simulink model "Distribution_v2"  (Simulink 7.9)
settings: Solver=VariableStepDiscrete  StartTime=0.0  StopTime=1000  RelTol=1e-3
libraries: simeventslib x35
(part 2 of 6)

== system Distribution_v2/Customer_6 ==
  Commodity_44 : Subsystem  mask{Mean=2000/49, AttributeValue=[6  18  22   1]|6|1|1}
      mask prompts: Mean "Frequency"; AttributeValue "Attributes"
  Commodity_45 : Subsystem  mask{Mean=2000/472, AttributeValue=[6  18   2   0]|6|2|1}
      mask prompts: Mean "Frequency"; AttributeValue "Attributes"
  Commodity_46 : Subsystem  mask{Mean=2000/118, AttributeValue=[6  18  22   5]|6|5|1}
      mask prompts: Mean "Frequency"; AttributeValue "Attributes"
  Commodity_47 : Subsystem  mask{Mean=2000/411, AttributeValue=[6  18  20   7]|6|7|1}
      mask prompts: Mean "Frequency"; AttributeValue "Attributes"
  Commodity_48 : Subsystem  mask{Mean=2000/22, AttributeValue=[6  18  20   8]|6|8|1}
      mask prompts: Mean "Frequency"; AttributeValue "Attributes"
  Commodity_49 : Subsystem  mask{Mean=2000/325, AttributeValue=[6  18   9   0]|6|9|1}
      mask prompts: Mean "Frequency"; AttributeValue "Attributes"
  Commodity_50 : Subsystem  mask{Mean=2000/274, AttributeValue=[6  18  22  12]|6|12|1}
      mask prompts: Mean "Frequency"; AttributeValue "Attributes"
  Commodity_51 : Subsystem  mask{Mean=2000/373, AttributeValue=[6  18  22  13]|6|13|1}
      mask prompts: Mean "Frequency"; AttributeValue "Attributes"
  Commodity_52 : Subsystem  mask{Mean=2000/344, AttributeValue=[6  18  20  14]|6|14|1}
      mask prompts: Mean "Frequency"; AttributeValue "Attributes"
  Commodity_53 : Subsystem  mask{Mean=2000/185, AttributeValue=[6  18  20  15]|6|15|1}
      mask prompts: Mean "Frequency"; AttributeValue "Attributes"
  Entity Sink : EntitySink
  Get Attribute : GetAttribute  AttributeName=Origin|Destination|Start  AttributeMissing=Error|Error|Error  AttributeDefaultValue=1|1|1  AttributeTreatAsVector=1|1|1  AttributeSendTiming=After entity departure|After entity departure|After entity departure  EvaluatedDefaultAttributeValue={[];[];[]}
      settings: OutputPortMap=o1,o2,o3
  Get Attribute1 : GetAttribute  AttributeName=Route  EvaluatedDefaultAttributeValue={[]}
      settings: OutputPortMap=o1
  IN_Commodity : PathCombiner  NumberInputPorts=10
  IN_Shipment : PathCombiner  NumberInputPorts=1
  Lookup : Constant  Value=[18]
  MATLAB Function : MATLAB Function  TreatAsAtomicUnit=on
  Mux : Mux  Inputs=3
  Node_ID : Constant  Value=6
  OUT_Shipment : OutputSwitch  NumberOutputPorts=1  SwitchingCriterion=From signal port p  AttributeName=Customer
  Shipment_Metrics : simeventslib/SimEvents Sinks/Discrete Event Signal to Workspace  VariableName=Customer_6  SaveFormat=Structure With Time  isMonitorOnly=off  isRecordIC=off
  Single Server : SingleServer  ServiceTime=0
  Timed to Evnt Signal : TimedToEventSignal
  Timed to Evnt Signal1 : TimedToEventSignal
  IN_Shipment_1 : PMIOPort  Port=1  Side=Left
  OUT_Shipment_1 : PMIOPort  Port=2  Side=Right
  wires:
  Timed to Evnt Signal1/1 -> MATLAB Function/3(lookup)
  Lookup/1 -> Timed to Evnt Signal1/1
  Timed to Evnt Signal/1 -> MATLAB Function/2(current)
  Get Attribute1/1 -> MATLAB Function/1(route)
  MATLAB Function/1(next) -> OUT_Shipment/1
  Node_ID/1 -> Timed to Evnt Signal/1
  Mux/1 -> Shipment_Metrics/1
  Get Attribute/3 -> Mux/3
  Get Attribute/2 -> Mux/2
  Get Attribute/1 -> Mux/1
  connections:
  Single Server/RConn1 -- OUT_Shipment/LConn1
  Get Attribute1/RConn1 -- Single Server/LConn1
  IN_Commodity/RConn1 -- Get Attribute1/LConn1
  Get Attribute/LConn1 -- IN_Shipment/RConn1
  Entity Sink/LConn1 -- Get Attribute/RConn1
  IN_Shipment/LConn1 -- IN_Shipment_1/RConn1
  OUT_Shipment/RConn1 -- OUT_Shipment_1/RConn1
  Commodity_44/RConn1 -- IN_Commodity/LConn1
  Commodity_45/RConn1 -- IN_Commodity/LConn2
  Commodity_46/RConn1 -- IN_Commodity/LConn3
  Commodity_47/RConn1 -- IN_Commodity/LConn4
  Commodity_48/RConn1 -- IN_Commodity/LConn5
  Commodity_49/RConn1 -- IN_Commodity/LConn6
  Commodity_50/RConn1 -- IN_Commodity/LConn7
  Commodity_51/RConn1 -- IN_Commodity/LConn8
  Commodity_52/RConn1 -- IN_Commodity/LConn9
  Commodity_53/RConn1 -- IN_Commodity/LConn10

== system Distribution_v2/Customer_7 ==
  Commodity_54 : Subsystem  mask{Mean=2000/465, AttributeValue=[7  20   3   0]|7|3|1}
      mask prompts: Mean "Frequency"; AttributeValue "Attributes"
  Commodity_55 : Subsystem  mask{Mean=2000/218, AttributeValue=[7  20  22   5]|7|5|1}
      mask prompts: Mean "Frequency"; AttributeValue "Attributes"
  Commodity_56 : Subsystem  mask{Mean=2000/154, AttributeValue=[7  20  18   6]|7|6|1}
      mask prompts: Mean "Frequency"; AttributeValue "Attributes"
  Commodity_57 : Subsystem  mask{Mean=2000/406, AttributeValue=[7  20  22  13]|7|13|1}
      mask prompts: Mean "Frequency"; AttributeValue "Attributes"
  Commodity_58 : Subsystem  mask{Mean=2000/470, AttributeValue=[7  20  15   0]|7|15|1}
      mask prompts: Mean "Frequency"; AttributeValue "Attributes"
  Entity Sink : EntitySink
  Get Attribute : GetAttribute  AttributeName=Origin|Destination|Start  AttributeMissing=Error|Error|Error  AttributeDefaultValue=1|1|1  AttributeTreatAsVector=1|1|1  AttributeSendTiming=After entity departure|After entity departure|After entity departure  EvaluatedDefaultAttributeValue={[];[];[]}
      settings: OutputPortMap=o1,o2,o3
  Get Attribute1 : GetAttribute  AttributeName=Route  EvaluatedDefaultAttributeValue={[]}
      settings: OutputPortMap=o1
  IN_Commodity : PathCombiner  NumberInputPorts=5
  IN_Shipment : PathCombiner  NumberInputPorts=1
  Lookup : Constant  Value=[20]
  MATLAB Function : MATLAB Function  TreatAsAtomicUnit=on
  Mux : Mux  Inputs=3
  Node_ID : Constant  Value=7
  OUT_Shipment : OutputSwitch  NumberOutputPorts=1  SwitchingCriterion=From signal port p  AttributeName=Customer
  Shipment_Metrics : simeventslib/SimEvents Sinks/Discrete Event Signal to Workspace  VariableName=Customer_7  SaveFormat=Structure With Time  isMonitorOnly=off  isRecordIC=off
  Single Server : SingleServer  ServiceTime=0
  Timed to Evnt Signal : TimedToEventSignal
  Timed to Evnt Signal1 : TimedToEventSignal
  IN_Shipment_1 : PMIOPort  Port=1  Side=Left
  OUT_Shipment_1 : PMIOPort  Port=2  Side=Right
  wires:
  Timed to Evnt Signal1/1 -> MATLAB Function/3(lookup)
  Lookup/1 -> Timed to Evnt Signal1/1
  Timed to Evnt Signal/1 -> MATLAB Function/2(current)
  Get Attribute1/1 -> MATLAB Function/1(route)
  MATLAB Function/1(next) -> OUT_Shipment/1
  Node_ID/1 -> Timed to Evnt Signal/1
  Mux/1 -> Shipment_Metrics/1
  Get Attribute/3 -> Mux/3
  Get Attribute/2 -> Mux/2
  Get Attribute/1 -> Mux/1
  connections:
  Single Server/RConn1 -- OUT_Shipment/LConn1
  Get Attribute1/RConn1 -- Single Server/LConn1
  IN_Commodity/RConn1 -- Get Attribute1/LConn1
  Get Attribute/LConn1 -- IN_Shipment/RConn1
  Entity Sink/LConn1 -- Get Attribute/RConn1
  IN_Shipment/LConn1 -- IN_Shipment_1/RConn1
  OUT_Shipment/RConn1 -- OUT_Shipment_1/RConn1
  Commodity_54/RConn1 -- IN_Commodity/LConn1
  Commodity_55/RConn1 -- IN_Commodity/LConn2
  Commodity_56/RConn1 -- IN_Commodity/LConn3
  Commodity_57/RConn1 -- IN_Commodity/LConn4
  Commodity_58/RConn1 -- IN_Commodity/LConn5

== system Distribution_v2/Customer_8 ==
  Commodity_59 : Subsystem  mask{Mean=2000/151, AttributeValue=[8  20  22   5]|8|5|1}
      mask prompts: Mean "Frequency"; AttributeValue "Attributes"
  Commodity_60 : Subsystem  mask{Mean=2000/116, AttributeValue=[8  20  18   6]|8|6|1}
      mask prompts: Mean "Frequency"; AttributeValue "Attributes"
  Commodity_61 : Subsystem  mask{Mean=2000/113, AttributeValue=[8  20  18   9]|8|9|1}
      mask prompts: Mean "Frequency"; AttributeValue "Attributes"
  Commodity_62 : Subsystem  mask{Mean=2000/114, AttributeValue=[8  20  22  10]|8|10|1}
      mask prompts: Mean "Frequency"; AttributeValue "Attributes"
  Commodity_63 : Subsystem  mask{Mean=2000/156, AttributeValue=[8  20  11   0]|8|11|1}
      mask prompts: Mean "Frequency"; AttributeValue "Attributes"
  Commodity_64 : Subsystem  mask{Mean=2000/93, AttributeValue=[8  20  22  13]|8|13|1}
      mask prompts: Mean "Frequency"; AttributeValue "Attributes"
  Entity Sink : EntitySink
  Get Attribute : GetAttribute  AttributeName=Origin|Destination|Start  AttributeMissing=Error|Error|Error  AttributeDefaultValue=1|1|1  AttributeTreatAsVector=1|1|1  AttributeSendTiming=After entity departure|After entity departure|After entity departure  EvaluatedDefaultAttributeValue={[];[];[]}
      settings: OutputPortMap=o1,o2,o3
  Get Attribute1 : GetAttribute  AttributeName=Route  EvaluatedDefaultAttributeValue={[]}
      settings: OutputPortMap=o1
  IN_Commodity : PathCombiner  NumberInputPorts=6
  IN_Shipment : PathCombiner  NumberInputPorts=1
  Lookup : Constant  Value=[20]
  MATLAB Function : MATLAB Function  TreatAsAtomicUnit=on
  Mux : Mux  Inputs=3
  Node_ID : Constant  Value=8
  OUT_Shipment : OutputSwitch  NumberOutputPorts=1  SwitchingCriterion=From signal port p  AttributeName=Customer
  Shipment_Metrics : simeventslib/SimEvents Sinks/Discrete Event Signal to Workspace  VariableName=Customer_8  SaveFormat=Structure With Time  isMonitorOnly=off  isRecordIC=off
  Single Server : SingleServer  ServiceTime=0
  Timed to Evnt Signal : TimedToEventSignal
  Timed to Evnt Signal1 : TimedToEventSignal
  IN_Shipment_1 : PMIOPort  Port=1  Side=Left
  OUT_Shipment_1 : PMIOPort  Port=2  Side=Right
  wires:
  Timed to Evnt Signal1/1 -> MATLAB Function/3(lookup)
  Lookup/1 -> Timed to Evnt Signal1/1
  Timed to Evnt Signal/1 -> MATLAB Function/2(current)
  Get Attribute1/1 -> MATLAB Function/1(route)
  MATLAB Function/1(next) -> OUT_Shipment/1
  Node_ID/1 -> Timed to Evnt Signal/1
  Mux/1 -> Shipment_Metrics/1
  Get Attribute/3 -> Mux/3
  Get Attribute/2 -> Mux/2
  Get Attribute/1 -> Mux/1
  connections:
  Single Server/RConn1 -- OUT_Shipment/LConn1
  Get Attribute1/RConn1 -- Single Server/LConn1
  IN_Commodity/RConn1 -- Get Attribute1/LConn1
  Get Attribute/LConn1 -- IN_Shipment/RConn1
  Entity Sink/LConn1 -- Get Attribute/RConn1
  IN_Shipment/LConn1 -- IN_Shipment_1/RConn1
  OUT_Shipment/RConn1 -- OUT_Shipment_1/RConn1
  Commodity_59/RConn1 -- IN_Commodity/LConn1
  Commodity_60/RConn1 -- IN_Commodity/LConn2
  Commodity_61/RConn1 -- IN_Commodity/LConn3
  Commodity_62/RConn1 -- IN_Commodity/LConn4
  Commodity_63/RConn1 -- IN_Commodity/LConn5
  Commodity_64/RConn1 -- IN_Commodity/LConn6

== system Distribution_v2/Customer_9 ==
  Commodity_65 : Subsystem  mask{Mean=2000/56, AttributeValue=[9  18  22   1]|9|1|1}
      mask prompts: Mean "Frequency"; AttributeValue "Attributes"
  Commodity_66 : Subsystem  mask{Mean=2000/205, AttributeValue=[9  18   2   0]|9|2|1}
      mask prompts: Mean "Frequency"; AttributeValue "Attributes"
  Commodity_67 : Subsystem  mask{Mean=2000/302, AttributeValue=[9  18   4   0]|9|4|1}
      mask prompts: Mean "Frequency"; AttributeValue "Attributes"
  Commodity_68 : Subsystem  mask{Mean=2000/59, AttributeValue=[9  18   6   0]|9|6|1}
      mask prompts: Mean "Frequency"; AttributeValue "Attributes"
  Commodity_69 : Subsystem  mask{Mean=2000/160, AttributeValue=[9  18  20   7]|9|7|1}
      mask prompts: Mean "Frequency"; AttributeValue "Attributes"
  Commodity_70 : Subsystem  mask{Mean=2000/254, AttributeValue=[9  18  20   8]|9|8|1}
      mask prompts: Mean "Frequency"; AttributeValue "Attributes"
  Commodity_71 : Subsystem  mask{Mean=2000/132, AttributeValue=[9  18  22  10]|9|10|1}
      mask prompts: Mean "Frequency"; AttributeValue "Attributes"
  Commodity_72 : Subsystem  mask{Mean=2000/465, AttributeValue=[9  18  22  12]|9|12|1}
      mask prompts: Mean "Frequency"; AttributeValue "Attributes"
  Commodity_73 : Subsystem  mask{Mean=2000/290, AttributeValue=[9  18  20  14]|9|14|1}
      mask prompts: Mean "Frequency"; AttributeValue "Attributes"
  Commodity_74 : Subsystem  mask{Mean=2000/230, AttributeValue=[9  18  20  15]|9|15|1}
      mask prompts: Mean "Frequency"; AttributeValue "Attributes"
  Entity Sink : EntitySink
  Get Attribute : GetAttribute  AttributeName=Origin|Destination|Start  AttributeMissing=Error|Error|Error  AttributeDefaultValue=1|1|1  AttributeTreatAsVector=1|1|1  AttributeSendTiming=After entity departure|After entity departure|After entity departure  EvaluatedDefaultAttributeValue={[];[];[]}
      settings: OutputPortMap=o1,o2,o3
  Get Attribute1 : GetAttribute  AttributeName=Route  EvaluatedDefaultAttributeValue={[]}
      settings: OutputPortMap=o1
  IN_Commodity : PathCombiner  NumberInputPorts=10
  IN_Shipment : PathCombiner  NumberInputPorts=1
  Lookup : Constant  Value=[18]
  MATLAB Function : MATLAB Function  TreatAsAtomicUnit=on
  Mux : Mux  Inputs=3
  Node_ID : Constant  Value=9
  OUT_Shipment : OutputSwitch  NumberOutputPorts=1  SwitchingCriterion=From signal port p  AttributeName=Customer
  Shipment_Metrics : simeventslib/SimEvents Sinks/Discrete Event Signal to Workspace  VariableName=Customer_9  SaveFormat=Structure With Time  isMonitorOnly=off  isRecordIC=off
  Single Server : SingleServer  ServiceTime=0
  Timed to Evnt Signal : TimedToEventSignal
  Timed to Evnt Signal1 : TimedToEventSignal
  IN_Shipment_1 : PMIOPort  Port=1  Side=Left
  OUT_Shipment_1 : PMIOPort  Port=2  Side=Right
  wires:
  Timed to Evnt Signal1/1 -> MATLAB Function/3(lookup)
  Lookup/1 -> Timed to Evnt Signal1/1
  Timed to Evnt Signal/1 -> MATLAB Function/2(current)
  Get Attribute1/1 -> MATLAB Function/1(route)
  MATLAB Function/1(next) -> OUT_Shipment/1
  Node_ID/1 -> Timed to Evnt Signal/1
  Mux/1 -> Shipment_Metrics/1
  Get Attribute/3 -> Mux/3
  Get Attribute/2 -> Mux/2
  Get Attribute/1 -> Mux/1
  connections:
  Single Server/RConn1 -- OUT_Shipment/LConn1
  Get Attribute1/RConn1 -- Single Server/LConn1
  IN_Commodity/RConn1 -- Get Attribute1/LConn1
  Get Attribute/LConn1 -- IN_Shipment/RConn1
  Entity Sink/LConn1 -- Get Attribute/RConn1
  IN_Shipment/LConn1 -- IN_Shipment_1/RConn1
  OUT_Shipment/RConn1 -- OUT_Shipment_1/RConn1
  Commodity_65/RConn1 -- IN_Commodity/LConn1
  Commodity_66/RConn1 -- IN_Commodity/LConn2
  Commodity_67/RConn1 -- IN_Commodity/LConn3
  Commodity_68/RConn1 -- IN_Commodity/LConn4
  Commodity_69/RConn1 -- IN_Commodity/LConn5
  Commodity_70/RConn1 -- IN_Commodity/LConn6
  Commodity_71/RConn1 -- IN_Commodity/LConn7
  Commodity_72/RConn1 -- IN_Commodity/LConn8
  Commodity_73/RConn1 -- IN_Commodity/LConn9
  Commodity_74/RConn1 -- IN_Commodity/LConn10

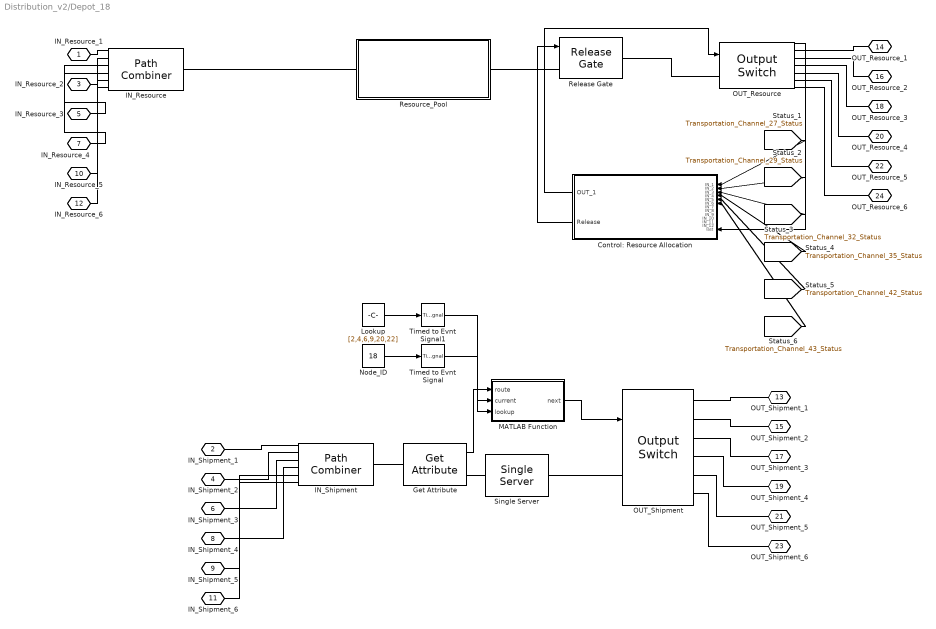
== system Distribution_v2/Depot_18 ==
  Control: Resource Allocation : MATLAB Function  TreatAsAtomicUnit=on
  Get Attribute : GetAttribute  AttributeName=Route  EvaluatedDefaultAttributeValue={[]}
      settings: OutputPortMap=o1
  IN_Resource : PathCombiner  NumberInputPorts=6
  IN_Shipment : PathCombiner  NumberInputPorts=6
  Lookup : Constant  Value=[2,4,6,9,20,22]
  MATLAB Function : MATLAB Function  TreatAsAtomicUnit=on
  Node_ID : Constant  Value=18
  OUT_Resource : OutputSwitch  NumberOutputPorts=6  SwitchingCriterion=From signal port p  InitialSeed=57769  StatLastDeparturePort=on
      settings: OutputPortMap=o3
  OUT_Shipment : OutputSwitch  NumberOutputPorts=6  SwitchingCriterion=From signal port p  AttributeName=Customer
  Release Gate : ReleaseGate  OpenGateUpon=Function call from port fcn
  Resource_Pool : Subsystem  mask{Quantity=6}
      mask prompts: Quantity "How many entities in resource pool?"
  Single Server : SingleServer  ServiceTime=0
  Timed to Evnt Signal : TimedToEventSignal
  Timed to Evnt Signal1 : TimedToEventSignal
  IN_Resource_1 : PMIOPort  Port=1  Side=Left
  IN_Shipment_1 : PMIOPort  Port=2  Side=Left
  IN_Resource_2 : PMIOPort  Port=3  Side=Left
  IN_Shipment_2 : PMIOPort  Port=4  Side=Left
  IN_Resource_3 : PMIOPort  Port=5  Side=Left
  IN_Shipment_3 : PMIOPort  Port=6  Side=Left
  IN_Resource_4 : PMIOPort  Port=7  Side=Left
  IN_Shipment_4 : PMIOPort  Port=8  Side=Left
  IN_Shipment_5 : PMIOPort  Port=9  Side=Left
  IN_Resource_5 : PMIOPort  Port=10  Side=Left
  IN_Shipment_6 : PMIOPort  Port=11  Side=Left
  IN_Resource_6 : PMIOPort  Port=12  Side=Left
  OUT_Shipment_1 : PMIOPort  Port=13  Side=Right
  OUT_Resource_1 : PMIOPort  Port=14  Side=Right
  OUT_Shipment_2 : PMIOPort  Port=15  Side=Right
  OUT_Resource_2 : PMIOPort  Port=16  Side=Right
  OUT_Shipment_3 : PMIOPort  Port=17  Side=Right
  OUT_Resource_3 : PMIOPort  Port=18  Side=Right
  OUT_Shipment_4 : PMIOPort  Port=19  Side=Right
  OUT_Resource_4 : PMIOPort  Port=20  Side=Right
  OUT_Shipment_5 : PMIOPort  Port=21  Side=Right
  OUT_Resource_5 : PMIOPort  Port=22  Side=Right
  OUT_Shipment_6 : PMIOPort  Port=23  Side=Right
  OUT_Resource_6 : PMIOPort  Port=24  Side=Right
  wires:
  OUT_Resource/1 -> Control: Resource Allocation/13(last)
  Control: Resource Allocation/2(Release) -> Release Gate/1
  Control: Resource Allocation/1(OUT_1) -> OUT_Resource/1
  Timed to Evnt Signal1/1 -> MATLAB Function/3(lookup)
  Lookup/1 -> Timed to Evnt Signal1/1
  Timed to Evnt Signal/1 -> MATLAB Function/2(current)
  Get Attribute/1 -> MATLAB Function/1(route)
  MATLAB Function/1(next) -> OUT_Shipment/1
  Node_ID/1 -> Timed to Evnt Signal/1
  [Transportation_Channel_27_Status] -> Control: Resource Allocation/1(IN_1)
  [Transportation_Channel_29_Status] -> Control: Resource Allocation/2(IN_2)
  [Transportation_Channel_32_Status] -> Control: Resource Allocation/3(IN_3)
  [Transportation_Channel_35_Status] -> Control: Resource Allocation/4(IN_4)
  [Transportation_Channel_42_Status] -> Control: Resource Allocation/5(IN_5)
  [Transportation_Channel_43_Status] -> Control: Resource Allocation/6(IN_6)
  connections:
  Release Gate/RConn1 -- OUT_Resource/LConn1
  Resource_Pool/LConn1 -- Release Gate/LConn1
  Single Server/RConn1 -- OUT_Shipment/LConn1
  Get Attribute/RConn1 -- Single Server/LConn1
  IN_Shipment/RConn1 -- Get Attribute/LConn1
  Resource_Pool/RConn1 -- IN_Resource/RConn1
  IN_Resource/LConn1 -- IN_Resource_1/RConn1
  IN_Resource/LConn2 -- IN_Resource_2/RConn1
  IN_Resource/LConn3 -- IN_Resource_3/RConn1
  IN_Resource/LConn4 -- IN_Resource_4/RConn1
  IN_Resource/LConn5 -- IN_Resource_5/RConn1
  IN_Resource/LConn6 -- IN_Resource_6/RConn1
  OUT_Resource/RConn1 -- OUT_Resource_1/RConn1
  OUT_Resource/RConn2 -- OUT_Resource_2/RConn1
  OUT_Resource/RConn3 -- OUT_Resource_3/RConn1
  OUT_Resource/RConn4 -- OUT_Resource_4/RConn1
  OUT_Resource/RConn5 -- OUT_Resource_5/RConn1
  OUT_Resource/RConn6 -- OUT_Resource_6/RConn1
  IN_Shipment/LConn1 -- IN_Shipment_1/RConn1
  IN_Shipment/LConn2 -- IN_Shipment_2/RConn1
  IN_Shipment/LConn3 -- IN_Shipment_3/RConn1
  IN_Shipment/LConn4 -- IN_Shipment_4/RConn1
  IN_Shipment/LConn5 -- IN_Shipment_5/RConn1
  IN_Shipment/LConn6 -- IN_Shipment_6/RConn1
  OUT_Shipment/RConn1 -- OUT_Shipment_1/RConn1
  OUT_Shipment/RConn2 -- OUT_Shipment_2/RConn1
  OUT_Shipment/RConn3 -- OUT_Shipment_3/RConn1
  OUT_Shipment/RConn4 -- OUT_Shipment_4/RConn1
  OUT_Shipment/RConn5 -- OUT_Shipment_5/RConn1
  OUT_Shipment/RConn6 -- OUT_Shipment_6/RConn1

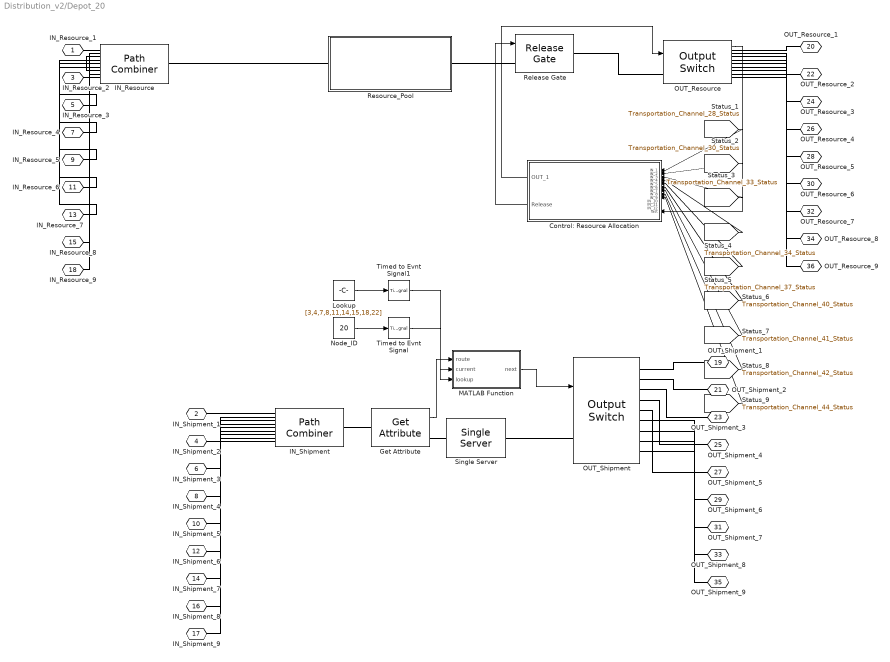
== system Distribution_v2/Depot_20 ==
  Control: Resource Allocation : MATLAB Function  TreatAsAtomicUnit=on
  Get Attribute : GetAttribute  AttributeName=Route  EvaluatedDefaultAttributeValue={[]}
      settings: OutputPortMap=o1
  IN_Resource : PathCombiner  NumberInputPorts=9
  IN_Shipment : PathCombiner  NumberInputPorts=9
  Lookup : Constant  Value=[3,4,7,8,11,14,15,18,22]
  MATLAB Function : MATLAB Function  TreatAsAtomicUnit=on
  Node_ID : Constant  Value=20
  OUT_Resource : OutputSwitch  NumberOutputPorts=9  SwitchingCriterion=From signal port p  InitialSeed=57769  StatLastDeparturePort=on
      settings: OutputPortMap=o3
  OUT_Shipment : OutputSwitch  NumberOutputPorts=9  SwitchingCriterion=From signal port p  AttributeName=Customer
  Release Gate : ReleaseGate  OpenGateUpon=Function call from port fcn
  Resource_Pool : Subsystem  mask{Quantity=6}
      mask prompts: Quantity "How many entities in resource pool?"
  Single Server : SingleServer  ServiceTime=0
  Timed to Evnt Signal : TimedToEventSignal
  Timed to Evnt Signal1 : TimedToEventSignal
  IN_Resource_1 : PMIOPort  Port=1  Side=Left
  IN_Shipment_1 : PMIOPort  Port=2  Side=Left
  IN_Resource_2 : PMIOPort  Port=3  Side=Left
  IN_Shipment_2 : PMIOPort  Port=4  Side=Left
  IN_Resource_3 : PMIOPort  Port=5  Side=Left
  IN_Shipment_3 : PMIOPort  Port=6  Side=Left
  IN_Resource_4 : PMIOPort  Port=7  Side=Left
  IN_Shipment_4 : PMIOPort  Port=8  Side=Left
  IN_Resource_5 : PMIOPort  Port=9  Side=Left
  IN_Shipment_5 : PMIOPort  Port=10  Side=Left
  IN_Resource_6 : PMIOPort  Port=11  Side=Left
  IN_Shipment_6 : PMIOPort  Port=12  Side=Left
  IN_Resource_7 : PMIOPort  Port=13  Side=Left
  IN_Shipment_7 : PMIOPort  Port=14  Side=Left
  IN_Resource_8 : PMIOPort  Port=15  Side=Left
  IN_Shipment_8 : PMIOPort  Port=16  Side=Left
  IN_Shipment_9 : PMIOPort  Port=17  Side=Left
  IN_Resource_9 : PMIOPort  Port=18  Side=Left
  OUT_Shipment_1 : PMIOPort  Port=19  Side=Right
  OUT_Resource_1 : PMIOPort  Port=20  Side=Right
  OUT_Shipment_2 : PMIOPort  Port=21  Side=Right
  OUT_Resource_2 : PMIOPort  Port=22  Side=Right
  OUT_Shipment_3 : PMIOPort  Port=23  Side=Right
  OUT_Resource_3 : PMIOPort  Port=24  Side=Right
  OUT_Shipment_4 : PMIOPort  Port=25  Side=Right
  OUT_Resource_4 : PMIOPort  Port=26  Side=Right
  OUT_Shipment_5 : PMIOPort  Port=27  Side=Right
  OUT_Resource_5 : PMIOPort  Port=28  Side=Right
  OUT_Shipment_6 : PMIOPort  Port=29  Side=Right
  OUT_Resource_6 : PMIOPort  Port=30  Side=Right
  OUT_Shipment_7 : PMIOPort  Port=31  Side=Right
  OUT_Resource_7 : PMIOPort  Port=32  Side=Right
  OUT_Shipment_8 : PMIOPort  Port=33  Side=Right
  OUT_Resource_8 : PMIOPort  Port=34  Side=Right
  OUT_Shipment_9 : PMIOPort  Port=35  Side=Right
  OUT_Resource_9 : PMIOPort  Port=36  Side=Right
  wires:
  OUT_Resource/1 -> Control: Resource Allocation/13(last)
  Control: Resource Allocation/2(Release) -> Release Gate/1
  Control: Resource Allocation/1(OUT_1) -> OUT_Resource/1
  Timed to Evnt Signal1/1 -> MATLAB Function/3(lookup)
  Lookup/1 -> Timed to Evnt Signal1/1
  Timed to Evnt Signal/1 -> MATLAB Function/2(current)
  Get Attribute/1 -> MATLAB Function/1(route)
  MATLAB Function/1(next) -> OUT_Shipment/1
  Node_ID/1 -> Timed to Evnt Signal/1
  [Transportation_Channel_28_Status] -> Control: Resource Allocation/1(IN_1)
  [Transportation_Channel_30_Status] -> Control: Resource Allocation/2(IN_2)
  [Transportation_Channel_33_Status] -> Control: Resource Allocation/3(IN_3)
  [Transportation_Channel_34_Status] -> Control: Resource Allocation/4(IN_4)
  [Transportation_Channel_37_Status] -> Control: Resource Allocation/5(IN_5)
  [Transportation_Channel_40_Status] -> Control: Resource Allocation/6(IN_6)
  [Transportation_Channel_41_Status] -> Control: Resource Allocation/7(IN_7)
  [Transportation_Channel_42_Status] -> Control: Resource Allocation/8(IN_8)
  [Transportation_Channel_44_Status] -> Control: Resource Allocation/9(IN_9)
  connections:
  Release Gate/RConn1 -- OUT_Resource/LConn1
  Resource_Pool/LConn1 -- Release Gate/LConn1
  Single Server/RConn1 -- OUT_Shipment/LConn1
  Get Attribute/RConn1 -- Single Server/LConn1
  IN_Shipment/RConn1 -- Get Attribute/LConn1
  Resource_Pool/RConn1 -- IN_Resource/RConn1
  IN_Resource/LConn1 -- IN_Resource_1/RConn1
  IN_Resource/LConn2 -- IN_Resource_2/RConn1
  IN_Resource/LConn3 -- IN_Resource_3/RConn1
  IN_Resource/LConn4 -- IN_Resource_4/RConn1
  IN_Resource/LConn5 -- IN_Resource_5/RConn1
  IN_Resource/LConn6 -- IN_Resource_6/RConn1
  IN_Resource/LConn7 -- IN_Resource_7/RConn1
  IN_Resource/LConn8 -- IN_Resource_8/RConn1
  IN_Resource/LConn9 -- IN_Resource_9/RConn1
  OUT_Resource/RConn1 -- OUT_Resource_1/RConn1
  OUT_Resource/RConn2 -- OUT_Resource_2/RConn1
  OUT_Resource/RConn3 -- OUT_Resource_3/RConn1
  OUT_Resource/RConn4 -- OUT_Resource_4/RConn1
  OUT_Resource/RConn5 -- OUT_Resource_5/RConn1
  OUT_Resource/RConn6 -- OUT_Resource_6/RConn1
  OUT_Resource/RConn7 -- OUT_Resource_7/RConn1
  OUT_Resource/RConn8 -- OUT_Resource_8/RConn1
  OUT_Resource/RConn9 -- OUT_Resource_9/RConn1
  IN_Shipment/LConn1 -- IN_Shipment_1/RConn1
  IN_Shipment/LConn2 -- IN_Shipment_2/RConn1
  IN_Shipment/LConn3 -- IN_Shipment_3/RConn1
  IN_Shipment/LConn4 -- IN_Shipment_4/RConn1
  IN_Shipment/LConn5 -- IN_Shipment_5/RConn1
  IN_Shipment/LConn6 -- IN_Shipment_6/RConn1
  IN_Shipment/LConn7 -- IN_Shipment_7/RConn1
  IN_Shipment/LConn8 -- IN_Shipment_8/RConn1
  IN_Shipment/LConn9 -- IN_Shipment_9/RConn1
  OUT_Shipment/RConn1 -- OUT_Shipment_1/RConn1
  OUT_Shipment/RConn2 -- OUT_Shipment_2/RConn1
  OUT_Shipment/RConn3 -- OUT_Shipment_3/RConn1
  OUT_Shipment/RConn4 -- OUT_Shipment_4/RConn1
  OUT_Shipment/RConn5 -- OUT_Shipment_5/RConn1
  OUT_Shipment/RConn6 -- OUT_Shipment_6/RConn1
  OUT_Shipment/RConn7 -- OUT_Shipment_7/RConn1
  OUT_Shipment/RConn8 -- OUT_Shipment_8/RConn1
  OUT_Shipment/RConn9 -- OUT_Shipment_9/RConn1

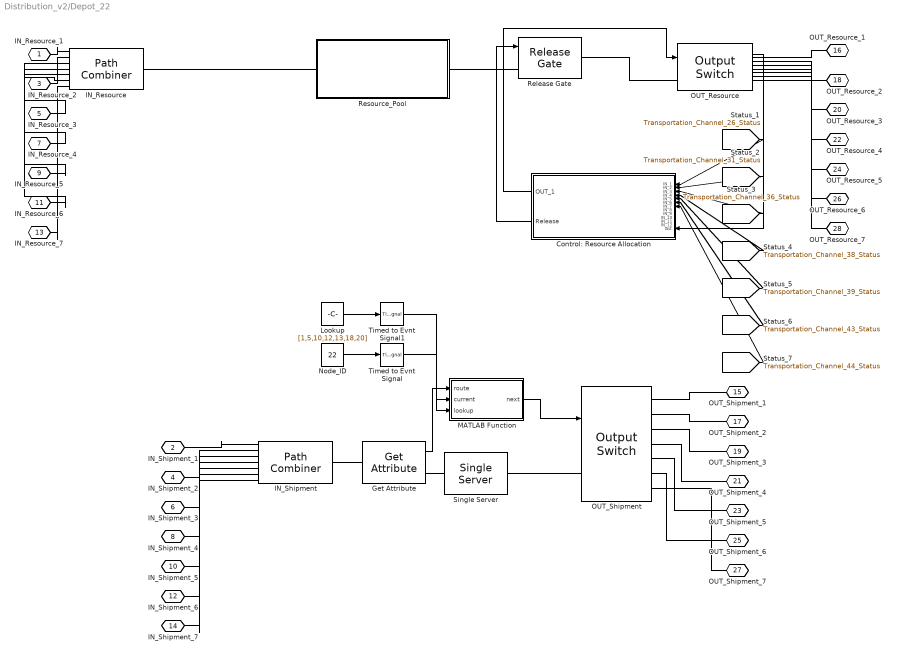
== system Distribution_v2/Depot_22 ==
  Control: Resource Allocation : MATLAB Function  TreatAsAtomicUnit=on
  Get Attribute : GetAttribute  AttributeName=Route  EvaluatedDefaultAttributeValue={[]}
      settings: OutputPortMap=o1
  IN_Resource : PathCombiner  NumberInputPorts=7
  IN_Shipment : PathCombiner  NumberInputPorts=7
  Lookup : Constant  Value=[1,5,10,12,13,18,20]
  MATLAB Function : MATLAB Function  TreatAsAtomicUnit=on
  Node_ID : Constant  Value=22
  OUT_Resource : OutputSwitch  NumberOutputPorts=7  SwitchingCriterion=From signal port p  InitialSeed=57769  StatLastDeparturePort=on
      settings: OutputPortMap=o3
  OUT_Shipment : OutputSwitch  NumberOutputPorts=7  SwitchingCriterion=From signal port p  AttributeName=Customer
  Release Gate : ReleaseGate  OpenGateUpon=Function call from port fcn
  Resource_Pool : Subsystem  mask{Quantity=6}
      mask prompts: Quantity "How many entities in resource pool?"
  Single Server : SingleServer  ServiceTime=0
  Timed to Evnt Signal : TimedToEventSignal
  Timed to Evnt Signal1 : TimedToEventSignal
  IN_Resource_1 : PMIOPort  Port=1  Side=Left
  IN_Shipment_1 : PMIOPort  Port=2  Side=Left
  IN_Resource_2 : PMIOPort  Port=3  Side=Left
  IN_Shipment_2 : PMIOPort  Port=4  Side=Left
  IN_Resource_3 : PMIOPort  Port=5  Side=Left
  IN_Shipment_3 : PMIOPort  Port=6  Side=Left
  IN_Resource_4 : PMIOPort  Port=7  Side=Left
  IN_Shipment_4 : PMIOPort  Port=8  Side=Left
  IN_Resource_5 : PMIOPort  Port=9  Side=Left
  IN_Shipment_5 : PMIOPort  Port=10  Side=Left
  IN_Resource_6 : PMIOPort  Port=11  Side=Left
  IN_Shipment_6 : PMIOPort  Port=12  Side=Left
  IN_Resource_7 : PMIOPort  Port=13  Side=Left
  IN_Shipment_7 : PMIOPort  Port=14  Side=Left
  OUT_Shipment_1 : PMIOPort  Port=15  Side=Right
  OUT_Resource_1 : PMIOPort  Port=16  Side=Right
  OUT_Shipment_2 : PMIOPort  Port=17  Side=Right
  OUT_Resource_2 : PMIOPort  Port=18  Side=Right
  OUT_Shipment_3 : PMIOPort  Port=19  Side=Right
  OUT_Resource_3 : PMIOPort  Port=20  Side=Right
  OUT_Shipment_4 : PMIOPort  Port=21  Side=Right
  OUT_Resource_4 : PMIOPort  Port=22  Side=Right
  OUT_Shipment_5 : PMIOPort  Port=23  Side=Right
  OUT_Resource_5 : PMIOPort  Port=24  Side=Right
  OUT_Shipment_6 : PMIOPort  Port=25  Side=Right
  OUT_Resource_6 : PMIOPort  Port=26  Side=Right
  OUT_Shipment_7 : PMIOPort  Port=27  Side=Right
  OUT_Resource_7 : PMIOPort  Port=28  Side=Right
  wires:
  OUT_Resource/1 -> Control: Resource Allocation/13(last)
  Control: Resource Allocation/2(Release) -> Release Gate/1
  Control: Resource Allocation/1(OUT_1) -> OUT_Resource/1
  Timed to Evnt Signal1/1 -> MATLAB Function/3(lookup)
  Lookup/1 -> Timed to Evnt Signal1/1
  Timed to Evnt Signal/1 -> MATLAB Function/2(current)
  Get Attribute/1 -> MATLAB Function/1(route)
  MATLAB Function/1(next) -> OUT_Shipment/1
  Node_ID/1 -> Timed to Evnt Signal/1
  [Transportation_Channel_26_Status] -> Control: Resource Allocation/1(IN_1)
  [Transportation_Channel_31_Status] -> Control: Resource Allocation/2(IN_2)
  [Transportation_Channel_36_Status] -> Control: Resource Allocation/3(IN_3)
  [Transportation_Channel_38_Status] -> Control: Resource Allocation/4(IN_4)
  [Transportation_Channel_39_Status] -> Control: Resource Allocation/5(IN_5)
  [Transportation_Channel_43_Status] -> Control: Resource Allocation/6(IN_6)
  [Transportation_Channel_44_Status] -> Control: Resource Allocation/7(IN_7)
  connections:
  Release Gate/RConn1 -- OUT_Resource/LConn1
  Resource_Pool/LConn1 -- Release Gate/LConn1
  Single Server/RConn1 -- OUT_Shipment/LConn1
  Get Attribute/RConn1 -- Single Server/LConn1
  IN_Shipment/RConn1 -- Get Attribute/LConn1
  Resource_Pool/RConn1 -- IN_Resource/RConn1
  IN_Resource/LConn1 -- IN_Resource_1/RConn1
  IN_Resource/LConn2 -- IN_Resource_2/RConn1
  IN_Resource/LConn3 -- IN_Resource_3/RConn1
  IN_Resource/LConn4 -- IN_Resource_4/RConn1
  IN_Resource/LConn5 -- IN_Resource_5/RConn1
  IN_Resource/LConn6 -- IN_Resource_6/RConn1
  IN_Resource/LConn7 -- IN_Resource_7/RConn1
  OUT_Resource/RConn1 -- OUT_Resource_1/RConn1
  OUT_Resource/RConn2 -- OUT_Resource_2/RConn1
  OUT_Resource/RConn3 -- OUT_Resource_3/RConn1
  OUT_Resource/RConn4 -- OUT_Resource_4/RConn1
  OUT_Resource/RConn5 -- OUT_Resource_5/RConn1
  OUT_Resource/RConn6 -- OUT_Resource_6/RConn1
  OUT_Resource/RConn7 -- OUT_Resource_7/RConn1
  IN_Shipment/LConn1 -- IN_Shipment_1/RConn1
  IN_Shipment/LConn2 -- IN_Shipment_2/RConn1
  IN_Shipment/LConn3 -- IN_Shipment_3/RConn1
  IN_Shipment/LConn4 -- IN_Shipment_4/RConn1
  IN_Shipment/LConn5 -- IN_Shipment_5/RConn1
  IN_Shipment/LConn6 -- IN_Shipment_6/RConn1
  IN_Shipment/LConn7 -- IN_Shipment_7/RConn1
  OUT_Shipment/RConn1 -- OUT_Shipment_1/RConn1
  OUT_Shipment/RConn2 -- OUT_Shipment_2/RConn1
  OUT_Shipment/RConn3 -- OUT_Shipment_3/RConn1
  OUT_Shipment/RConn4 -- OUT_Shipment_4/RConn1
  OUT_Shipment/RConn5 -- OUT_Shipment_5/RConn1
  OUT_Shipment/RConn6 -- OUT_Shipment_6/RConn1
  OUT_Shipment/RConn7 -- OUT_Shipment_7/RConn1

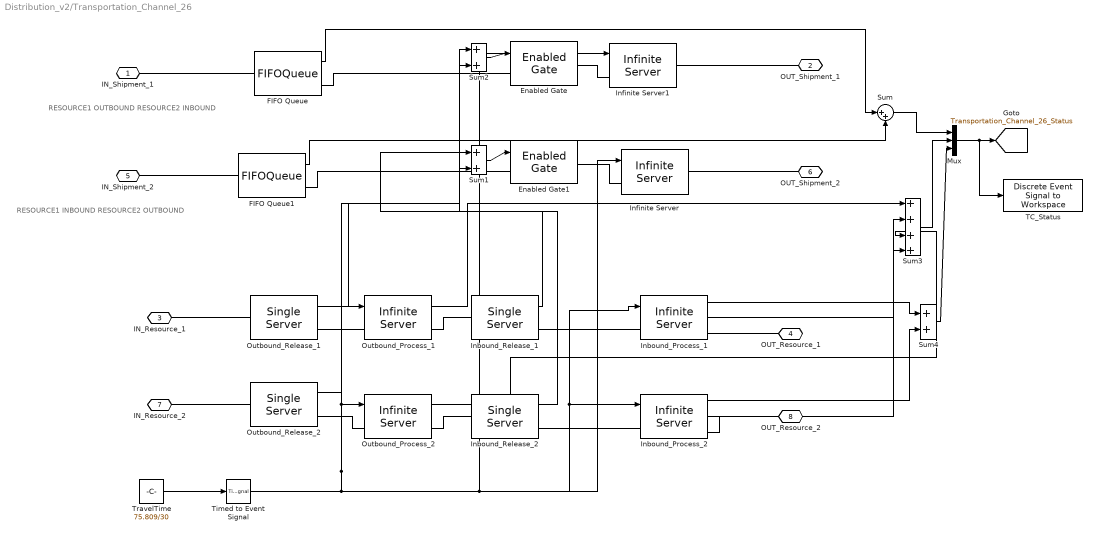
== system Distribution_v2/Transportation_Channel_26 ==
  note: RESOURCE1 OUTBOUND
      | RESOURCE2 INBOUND
  note: RESOURCE1 INBOUND
      | RESOURCE2 OUTBOUND
  Enabled Gate : EnabledGate
  Enabled Gate1 : EnabledGate
  FIFO Queue : FIFOQueue  Capacity=inf  StatNumberInBlock=on
      settings: OutputPortMap=o1
  FIFO Queue1 : FIFOQueue  Capacity=inf  StatNumberInBlock=on
      settings: OutputPortMap=o1
  Inbound_Process_1 : InfiniteServer  ServiceTimeFrom=Signal port t  ServiceTime=(76.7)/30  StatNumberDeparted=on  StatNumberInBlock=on
      settings: OutputPortMap=o0,o1
  Inbound_Process_2 : InfiniteServer  ServiceTimeFrom=Signal port t  ServiceTime=(76.7)/30  StatNumberDeparted=on  StatNumberInBlock=on
      settings: OutputPortMap=o0,o1
  Inbound_Release_1 : SingleServer  ServiceTime=0  StatNumberInBlock=on
      settings: OutputPortMap=o1
  Inbound_Release_2 : SingleServer  ServiceTime=0  StatNumberInBlock=on
      settings: OutputPortMap=o1
  Infinite Server : InfiniteServer  ServiceTimeFrom=Signal port t  ServiceTime=(76.7)/30
  Infinite Server1 : InfiniteServer  ServiceTimeFrom=Signal port t  ServiceTime=(76.7)/30
  Mux : Mux  Inputs=3
  Outbound_Process_1 : InfiniteServer  ServiceTimeFrom=Signal port t  ServiceTime=(76.7)/30  StatNumberInBlock=on
      settings: OutputPortMap=o1
  Outbound_Process_2 : InfiniteServer  ServiceTimeFrom=Signal port t  ServiceTime=(76.7)/30  StatNumberInBlock=on
      settings: OutputPortMap=o1
  Outbound_Release_1 : SingleServer  ServiceTime=0  StatNumberInBlock=on
      settings: OutputPortMap=o1
  Outbound_Release_2 : SingleServer  ServiceTime=0  StatNumberInBlock=on
      settings: OutputPortMap=o1
  Sum{,1..2,4} (4 alike) : Sum  Inputs=|++
  Sum3 : Sum  Inputs=|++++
  TC_Status : simeventslib/SimEvents Sinks/Discrete Event Signal to Workspace  VariableName=Transportation_Channel_26_Status  SaveFormat=Structure With Time  isMonitorOnly=off  isRecordIC=off
  Timed to Event Signal : TimedToEventSignal
  TravelTime : Constant  Value=75.809/30
  IN_Shipment_1 : PMIOPort  Port=1  Side=Left
  OUT_Shipment_1 : PMIOPort  Port=2  Side=Right
  IN_Resource_1 : PMIOPort  Port=3  Side=Left
  OUT_Resource_1 : PMIOPort  Port=4  Side=Right
  IN_Shipment_2 : PMIOPort  Port=5  Side=Left
  OUT_Shipment_2 : PMIOPort  Port=6  Side=Right
  IN_Resource_2 : PMIOPort  Port=7  Side=Left
  OUT_Resource_2 : PMIOPort  Port=8  Side=Right
  tag scope: Transportation_Channel_26_Status=global
  wires:
  Sum4/1 -> Mux/3
  Inbound_Process_2/1 -> Sum4/2
  Inbound_Process_1/1 -> Sum4/1
  Inbound_Process_2/2 -> Sum3/4
  Outbound_Process_2/1 -> Sum3/3
  Inbound_Process_1/2 -> Sum3/2
  Outbound_Process_1/1 -> Sum3/1
  Sum3/1 -> Mux/2
  Sum/1 -> Mux/1
  Mux/1 -> TC_Status/1, [Transportation_Channel_26_Status]
  Inbound_Release_2/1 -> Sum2/2
  Outbound_Release_1/1 -> Sum2/1
  Sum2/1 -> Enabled Gate/1
  Inbound_Release_1/1 -> Sum1/1
  Outbound_Release_2/1 -> Sum1/2
  Sum1/1 -> Enabled Gate1/1
  Timed to Event Signal/1 -> Infinite Server/1, Inbound_Process_2/1, Inbound_Process_1/1, Infinite Server1/1, Outbound_Process_2/1, Outbound_Process_1/1
  TravelTime/1 -> Timed to Event Signal/1
  FIFO Queue/1 -> Sum/1
  FIFO Queue1/1 -> Sum/2
  connections:
  Inbound_Process_1/RConn1 -- OUT_Resource_1/RConn1
  Outbound_Process_1/RConn1 -- Inbound_Release_1/LConn1
  Inbound_Release_1/RConn1 -- Inbound_Process_1/LConn1
  Outbound_Release_1/RConn1 -- Outbound_Process_1/LConn1
  Inbound_Process_2/RConn1 -- OUT_Resource_2/RConn1
  Inbound_Release_2/RConn1 -- Inbound_Process_2/LConn1
  Outbound_Process_2/RConn1 -- Inbound_Release_2/LConn1
  Outbound_Release_2/RConn1 -- Outbound_Process_2/LConn1
  IN_Resource_2/RConn1 -- Outbound_Release_2/LConn1
  Infinite Server1/RConn1 -- OUT_Shipment_1/RConn1
  Enabled Gate/RConn1 -- Infinite Server1/LConn1
  Infinite Server/LConn1 -- Enabled Gate1/RConn1
  OUT_Shipment_2/RConn1 -- Infinite Server/RConn1
  IN_Resource_1/RConn1 -- Outbound_Release_1/LConn1
  IN_Shipment_2/RConn1 -- FIFO Queue1/LConn1
  IN_Shipment_1/RConn1 -- FIFO Queue/LConn1
  Enabled Gate1/LConn1 -- FIFO Queue1/RConn1
  FIFO Queue/RConn1 -- Enabled Gate/LConn1

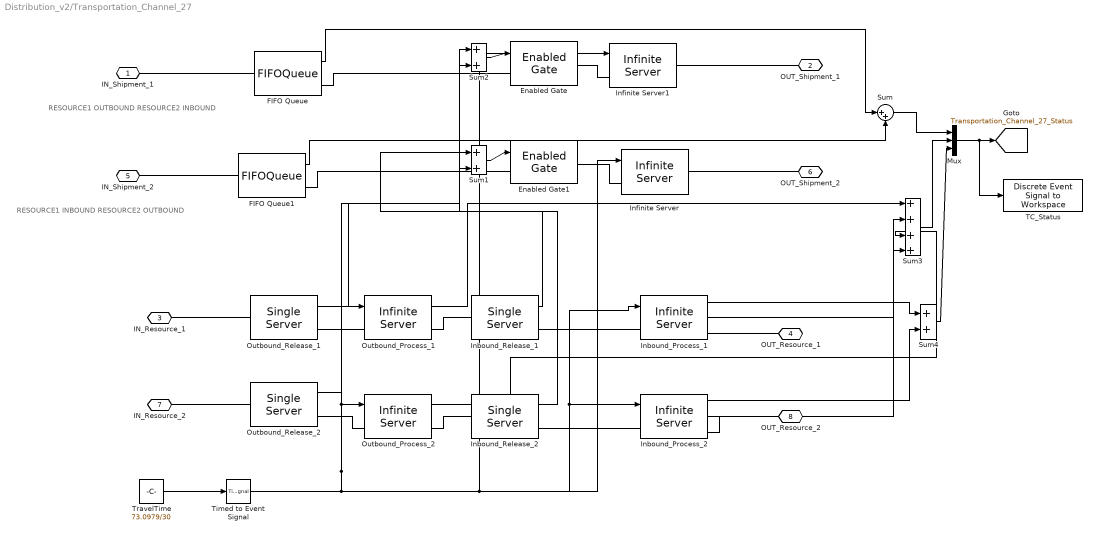
== system Distribution_v2/Transportation_Channel_27 ==
  note: RESOURCE1 OUTBOUND
      | RESOURCE2 INBOUND
  note: RESOURCE1 INBOUND
      | RESOURCE2 OUTBOUND
  Enabled Gate : EnabledGate
  Enabled Gate1 : EnabledGate
  FIFO Queue : FIFOQueue  Capacity=inf  StatNumberInBlock=on
      settings: OutputPortMap=o1
  FIFO Queue1 : FIFOQueue  Capacity=inf  StatNumberInBlock=on
      settings: OutputPortMap=o1
  Inbound_Process_1 : InfiniteServer  ServiceTimeFrom=Signal port t  ServiceTime=(76.7)/30  StatNumberDeparted=on  StatNumberInBlock=on
      settings: OutputPortMap=o0,o1
  Inbound_Process_2 : InfiniteServer  ServiceTimeFrom=Signal port t  ServiceTime=(76.7)/30  StatNumberDeparted=on  StatNumberInBlock=on
      settings: OutputPortMap=o0,o1
  Inbound_Release_1 : SingleServer  ServiceTime=0  StatNumberInBlock=on
      settings: OutputPortMap=o1
  Inbound_Release_2 : SingleServer  ServiceTime=0  StatNumberInBlock=on
      settings: OutputPortMap=o1
  Infinite Server : InfiniteServer  ServiceTimeFrom=Signal port t  ServiceTime=(76.7)/30
  Infinite Server1 : InfiniteServer  ServiceTimeFrom=Signal port t  ServiceTime=(76.7)/30
  Mux : Mux  Inputs=3
  Outbound_Process_1 : InfiniteServer  ServiceTimeFrom=Signal port t  ServiceTime=(76.7)/30  StatNumberInBlock=on
      settings: OutputPortMap=o1
  Outbound_Process_2 : InfiniteServer  ServiceTimeFrom=Signal port t  ServiceTime=(76.7)/30  StatNumberInBlock=on
      settings: OutputPortMap=o1
  Outbound_Release_1 : SingleServer  ServiceTime=0  StatNumberInBlock=on
      settings: OutputPortMap=o1
  Outbound_Release_2 : SingleServer  ServiceTime=0  StatNumberInBlock=on
      settings: OutputPortMap=o1
  Sum{,1..2,4} (4 alike) : Sum  Inputs=|++
  Sum3 : Sum  Inputs=|++++
  TC_Status : simeventslib/SimEvents Sinks/Discrete Event Signal to Workspace  VariableName=Transportation_Channel_27_Status  SaveFormat=Structure With Time  isMonitorOnly=off  isRecordIC=off
  Timed to Event Signal : TimedToEventSignal
  TravelTime : Constant  Value=73.0979/30
  IN_Shipment_1 : PMIOPort  Port=1  Side=Left
  OUT_Shipment_1 : PMIOPort  Port=2  Side=Right
  IN_Resource_1 : PMIOPort  Port=3  Side=Left
  OUT_Resource_1 : PMIOPort  Port=4  Side=Right
  IN_Shipment_2 : PMIOPort  Port=5  Side=Left
  OUT_Shipment_2 : PMIOPort  Port=6  Side=Right
  IN_Resource_2 : PMIOPort  Port=7  Side=Left
  OUT_Resource_2 : PMIOPort  Port=8  Side=Right
  tag scope: Transportation_Channel_27_Status=global
  wires:
  Sum4/1 -> Mux/3
  Inbound_Process_2/1 -> Sum4/2
  Inbound_Process_1/1 -> Sum4/1
  Inbound_Process_2/2 -> Sum3/4
  Outbound_Process_2/1 -> Sum3/3
  Inbound_Process_1/2 -> Sum3/2
  Outbound_Process_1/1 -> Sum3/1
  Sum3/1 -> Mux/2
  Sum/1 -> Mux/1
  Mux/1 -> TC_Status/1, [Transportation_Channel_27_Status]
  Inbound_Release_2/1 -> Sum2/2
  Outbound_Release_1/1 -> Sum2/1
  Sum2/1 -> Enabled Gate/1
  Inbound_Release_1/1 -> Sum1/1
  Outbound_Release_2/1 -> Sum1/2
  Sum1/1 -> Enabled Gate1/1
  Timed to Event Signal/1 -> Infinite Server/1, Inbound_Process_2/1, Inbound_Process_1/1, Infinite Server1/1, Outbound_Process_2/1, Outbound_Process_1/1
  TravelTime/1 -> Timed to Event Signal/1
  FIFO Queue/1 -> Sum/1
  FIFO Queue1/1 -> Sum/2
  connections:
  Inbound_Process_1/RConn1 -- OUT_Resource_1/RConn1
  Outbound_Process_1/RConn1 -- Inbound_Release_1/LConn1
  Inbound_Release_1/RConn1 -- Inbound_Process_1/LConn1
  Outbound_Release_1/RConn1 -- Outbound_Process_1/LConn1
  Inbound_Process_2/RConn1 -- OUT_Resource_2/RConn1
  Inbound_Release_2/RConn1 -- Inbound_Process_2/LConn1
  Outbound_Process_2/RConn1 -- Inbound_Release_2/LConn1
  Outbound_Release_2/RConn1 -- Outbound_Process_2/LConn1
  IN_Resource_2/RConn1 -- Outbound_Release_2/LConn1
  Infinite Server1/RConn1 -- OUT_Shipment_1/RConn1
  Enabled Gate/RConn1 -- Infinite Server1/LConn1
  Infinite Server/LConn1 -- Enabled Gate1/RConn1
  OUT_Shipment_2/RConn1 -- Infinite Server/RConn1
  IN_Resource_1/RConn1 -- Outbound_Release_1/LConn1
  IN_Shipment_2/RConn1 -- FIFO Queue1/LConn1
  IN_Shipment_1/RConn1 -- FIFO Queue/LConn1
  Enabled Gate1/LConn1 -- FIFO Queue1/RConn1
  FIFO Queue/RConn1 -- Enabled Gate/LConn1

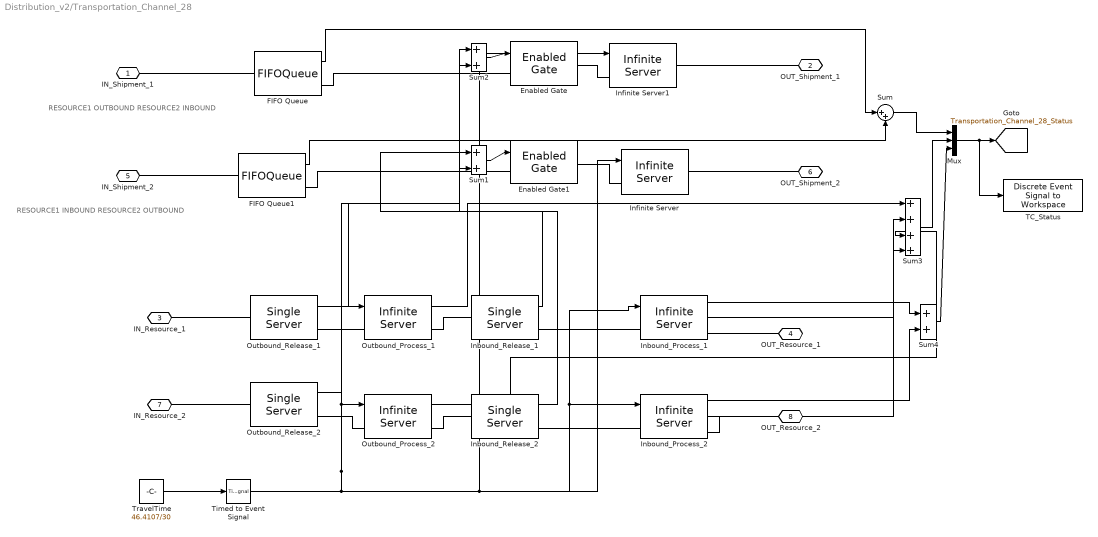
== system Distribution_v2/Transportation_Channel_28 ==
  note: RESOURCE1 OUTBOUND
      | RESOURCE2 INBOUND
  note: RESOURCE1 INBOUND
      | RESOURCE2 OUTBOUND
  Enabled Gate : EnabledGate
  Enabled Gate1 : EnabledGate
  FIFO Queue : FIFOQueue  Capacity=inf  StatNumberInBlock=on
      settings: OutputPortMap=o1
  FIFO Queue1 : FIFOQueue  Capacity=inf  StatNumberInBlock=on
      settings: OutputPortMap=o1
  Inbound_Process_1 : InfiniteServer  ServiceTimeFrom=Signal port t  ServiceTime=(76.7)/30  StatNumberDeparted=on  StatNumberInBlock=on
      settings: OutputPortMap=o0,o1
  Inbound_Process_2 : InfiniteServer  ServiceTimeFrom=Signal port t  ServiceTime=(76.7)/30  StatNumberDeparted=on  StatNumberInBlock=on
      settings: OutputPortMap=o0,o1
  Inbound_Release_1 : SingleServer  ServiceTime=0  StatNumberInBlock=on
      settings: OutputPortMap=o1
  Inbound_Release_2 : SingleServer  ServiceTime=0  StatNumberInBlock=on
      settings: OutputPortMap=o1
  Infinite Server : InfiniteServer  ServiceTimeFrom=Signal port t  ServiceTime=(76.7)/30
  Infinite Server1 : InfiniteServer  ServiceTimeFrom=Signal port t  ServiceTime=(76.7)/30
  Mux : Mux  Inputs=3
  Outbound_Process_1 : InfiniteServer  ServiceTimeFrom=Signal port t  ServiceTime=(76.7)/30  StatNumberInBlock=on
      settings: OutputPortMap=o1
  Outbound_Process_2 : InfiniteServer  ServiceTimeFrom=Signal port t  ServiceTime=(76.7)/30  StatNumberInBlock=on
      settings: OutputPortMap=o1
  Outbound_Release_1 : SingleServer  ServiceTime=0  StatNumberInBlock=on
      settings: OutputPortMap=o1
  Outbound_Release_2 : SingleServer  ServiceTime=0  StatNumberInBlock=on
      settings: OutputPortMap=o1
  Sum{,1..2,4} (4 alike) : Sum  Inputs=|++
  Sum3 : Sum  Inputs=|++++
  TC_Status : simeventslib/SimEvents Sinks/Discrete Event Signal to Workspace  VariableName=Transportation_Channel_28_Status  SaveFormat=Structure With Time  isMonitorOnly=off  isRecordIC=off
  Timed to Event Signal : TimedToEventSignal
  TravelTime : Constant  Value=46.4107/30
  IN_Shipment_1 : PMIOPort  Port=1  Side=Left
  OUT_Shipment_1 : PMIOPort  Port=2  Side=Right
  IN_Resource_1 : PMIOPort  Port=3  Side=Left
  OUT_Resource_1 : PMIOPort  Port=4  Side=Right
  IN_Shipment_2 : PMIOPort  Port=5  Side=Left
  OUT_Shipment_2 : PMIOPort  Port=6  Side=Right
  IN_Resource_2 : PMIOPort  Port=7  Side=Left
  OUT_Resource_2 : PMIOPort  Port=8  Side=Right
  tag scope: Transportation_Channel_28_Status=global
  wires:
  Sum4/1 -> Mux/3
  Inbound_Process_2/1 -> Sum4/2
  Inbound_Process_1/1 -> Sum4/1
  Inbound_Process_2/2 -> Sum3/4
  Outbound_Process_2/1 -> Sum3/3
  Inbound_Process_1/2 -> Sum3/2
  Outbound_Process_1/1 -> Sum3/1
  Sum3/1 -> Mux/2
  Sum/1 -> Mux/1
  Mux/1 -> TC_Status/1, [Transportation_Channel_28_Status]
  Inbound_Release_2/1 -> Sum2/2
  Outbound_Release_1/1 -> Sum2/1
  Sum2/1 -> Enabled Gate/1
  Inbound_Release_1/1 -> Sum1/1
  Outbound_Release_2/1 -> Sum1/2
  Sum1/1 -> Enabled Gate1/1
  Timed to Event Signal/1 -> Infinite Server/1, Inbound_Process_2/1, Inbound_Process_1/1, Infinite Server1/1, Outbound_Process_2/1, Outbound_Process_1/1
  TravelTime/1 -> Timed to Event Signal/1
  FIFO Queue/1 -> Sum/1
  FIFO Queue1/1 -> Sum/2
  connections:
  Inbound_Process_1/RConn1 -- OUT_Resource_1/RConn1
  Outbound_Process_1/RConn1 -- Inbound_Release_1/LConn1
  Inbound_Release_1/RConn1 -- Inbound_Process_1/LConn1
  Outbound_Release_1/RConn1 -- Outbound_Process_1/LConn1
  Inbound_Process_2/RConn1 -- OUT_Resource_2/RConn1
  Inbound_Release_2/RConn1 -- Inbound_Process_2/LConn1
  Outbound_Process_2/RConn1 -- Inbound_Release_2/LConn1
  Outbound_Release_2/RConn1 -- Outbound_Process_2/LConn1
  IN_Resource_2/RConn1 -- Outbound_Release_2/LConn1
  Infinite Server1/RConn1 -- OUT_Shipment_1/RConn1
  Enabled Gate/RConn1 -- Infinite Server1/LConn1
  Infinite Server/LConn1 -- Enabled Gate1/RConn1
  OUT_Shipment_2/RConn1 -- Infinite Server/RConn1
  IN_Resource_1/RConn1 -- Outbound_Release_1/LConn1
  IN_Shipment_2/RConn1 -- FIFO Queue1/LConn1
  IN_Shipment_1/RConn1 -- FIFO Queue/LConn1
  Enabled Gate1/LConn1 -- FIFO Queue1/RConn1
  FIFO Queue/RConn1 -- Enabled Gate/LConn1

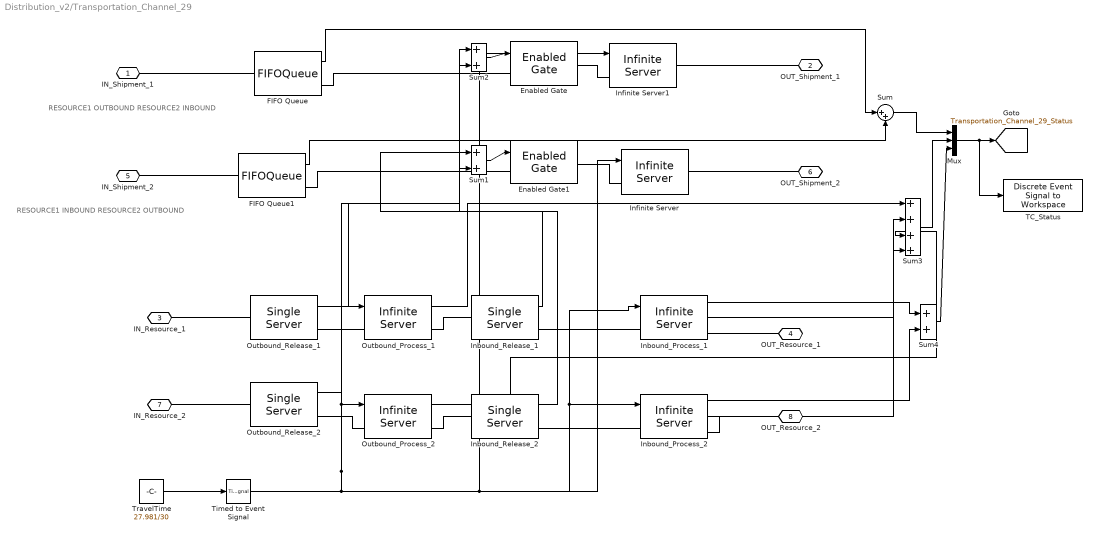
== system Distribution_v2/Transportation_Channel_29 ==
  note: RESOURCE1 OUTBOUND
      | RESOURCE2 INBOUND
  note: RESOURCE1 INBOUND
      | RESOURCE2 OUTBOUND
  Enabled Gate : EnabledGate
  Enabled Gate1 : EnabledGate
  FIFO Queue : FIFOQueue  Capacity=inf  StatNumberInBlock=on
      settings: OutputPortMap=o1
  FIFO Queue1 : FIFOQueue  Capacity=inf  StatNumberInBlock=on
      settings: OutputPortMap=o1
  Inbound_Process_1 : InfiniteServer  ServiceTimeFrom=Signal port t  ServiceTime=(76.7)/30  StatNumberDeparted=on  StatNumberInBlock=on
      settings: OutputPortMap=o0,o1
  Inbound_Process_2 : InfiniteServer  ServiceTimeFrom=Signal port t  ServiceTime=(76.7)/30  StatNumberDeparted=on  StatNumberInBlock=on
      settings: OutputPortMap=o0,o1
  Inbound_Release_1 : SingleServer  ServiceTime=0  StatNumberInBlock=on
      settings: OutputPortMap=o1
  Inbound_Release_2 : SingleServer  ServiceTime=0  StatNumberInBlock=on
      settings: OutputPortMap=o1
  Infinite Server : InfiniteServer  ServiceTimeFrom=Signal port t  ServiceTime=(76.7)/30
  Infinite Server1 : InfiniteServer  ServiceTimeFrom=Signal port t  ServiceTime=(76.7)/30
  Mux : Mux  Inputs=3
  Outbound_Process_1 : InfiniteServer  ServiceTimeFrom=Signal port t  ServiceTime=(76.7)/30  StatNumberInBlock=on
      settings: OutputPortMap=o1
  Outbound_Process_2 : InfiniteServer  ServiceTimeFrom=Signal port t  ServiceTime=(76.7)/30  StatNumberInBlock=on
      settings: OutputPortMap=o1
  Outbound_Release_1 : SingleServer  ServiceTime=0  StatNumberInBlock=on
      settings: OutputPortMap=o1
  Outbound_Release_2 : SingleServer  ServiceTime=0  StatNumberInBlock=on
      settings: OutputPortMap=o1
  Sum{,1..2,4} (4 alike) : Sum  Inputs=|++
  Sum3 : Sum  Inputs=|++++
  TC_Status : simeventslib/SimEvents Sinks/Discrete Event Signal to Workspace  VariableName=Transportation_Channel_29_Status  SaveFormat=Structure With Time  isMonitorOnly=off  isRecordIC=off
  Timed to Event Signal : TimedToEventSignal
  TravelTime : Constant  Value=27.981/30
  IN_Shipment_1 : PMIOPort  Port=1  Side=Left
  OUT_Shipment_1 : PMIOPort  Port=2  Side=Right
  IN_Resource_1 : PMIOPort  Port=3  Side=Left
  OUT_Resource_1 : PMIOPort  Port=4  Side=Right
  IN_Shipment_2 : PMIOPort  Port=5  Side=Left
  OUT_Shipment_2 : PMIOPort  Port=6  Side=Right
  IN_Resource_2 : PMIOPort  Port=7  Side=Left
  OUT_Resource_2 : PMIOPort  Port=8  Side=Right
  tag scope: Transportation_Channel_29_Status=global
  wires:
  Sum4/1 -> Mux/3
  Inbound_Process_2/1 -> Sum4/2
  Inbound_Process_1/1 -> Sum4/1
  Inbound_Process_2/2 -> Sum3/4
  Outbound_Process_2/1 -> Sum3/3
  Inbound_Process_1/2 -> Sum3/2
  Outbound_Process_1/1 -> Sum3/1
  Sum3/1 -> Mux/2
  Sum/1 -> Mux/1
  Mux/1 -> TC_Status/1, [Transportation_Channel_29_Status]
  Inbound_Release_2/1 -> Sum2/2
  Outbound_Release_1/1 -> Sum2/1
  Sum2/1 -> Enabled Gate/1
  Inbound_Release_1/1 -> Sum1/1
  Outbound_Release_2/1 -> Sum1/2
  Sum1/1 -> Enabled Gate1/1
  Timed to Event Signal/1 -> Infinite Server/1, Inbound_Process_2/1, Inbound_Process_1/1, Infinite Server1/1, Outbound_Process_2/1, Outbound_Process_1/1
  TravelTime/1 -> Timed to Event Signal/1
  FIFO Queue/1 -> Sum/1
  FIFO Queue1/1 -> Sum/2
  connections:
  Inbound_Process_1/RConn1 -- OUT_Resource_1/RConn1
  Outbound_Process_1/RConn1 -- Inbound_Release_1/LConn1
  Inbound_Release_1/RConn1 -- Inbound_Process_1/LConn1
  Outbound_Release_1/RConn1 -- Outbound_Process_1/LConn1
  Inbound_Process_2/RConn1 -- OUT_Resource_2/RConn1
  Inbound_Release_2/RConn1 -- Inbound_Process_2/LConn1
  Outbound_Process_2/RConn1 -- Inbound_Release_2/LConn1
  Outbound_Release_2/RConn1 -- Outbound_Process_2/LConn1
  IN_Resource_2/RConn1 -- Outbound_Release_2/LConn1
  Infinite Server1/RConn1 -- OUT_Shipment_1/RConn1
  Enabled Gate/RConn1 -- Infinite Server1/LConn1
  Infinite Server/LConn1 -- Enabled Gate1/RConn1
  OUT_Shipment_2/RConn1 -- Infinite Server/RConn1
  IN_Resource_1/RConn1 -- Outbound_Release_1/LConn1
  IN_Shipment_2/RConn1 -- FIFO Queue1/LConn1
  IN_Shipment_1/RConn1 -- FIFO Queue/LConn1
  Enabled Gate1/LConn1 -- FIFO Queue1/RConn1
  FIFO Queue/RConn1 -- Enabled Gate/LConn1
